simulink model "I_f_control_Rotor_pos_est"  (R2021b)
settings: Solver=FixedStepDiscrete  StartTime=0.0  StopTime=inf  RelTol=1e-3  EnableMultiTasking=on
model workspace (MAT data in the model file):
  samples = 1000
values from neighbouring files (symbols this model uses):
  alphac = 2*pi*300    (= 1884.95559215)    [init.m]
  Ls = 0.2e-3    (= 0.0002)    [init.m]
  max_rate = 100    [init.m]
  min_rate = -100    [init.m]
  p = 8    [Mtpa.m]    (also in init.m = 4)
  PositionOffset = 3.512    [init.m]
  psi_f = single((Ke)/(sqrt(3)*2*pi*1000*p/60))    [init.m]
  PWM_timer_period = (CPU_clock/Sys_clock_div/fsw/2)/4    (= 1250)    [init.m]
  Rs = 0.36    [init.m]
  Time_needed = Timeconstant*5    (= 0.00277777777778)    [init.m]
  Ts = 1/(4*fsw)    (= 2.5e-05)    [init.m]
undefined symbols (not defined in the file or in its folder): Down, GPTRIP1SEL, GPTRIP2SEL, TZ1, TZ2, Up
libraries: c2802xlib x7, c280xlib x3, c2837xDlib x3, mcbpositiondecoderlib x3, c2000lib x1, simulink x1
(part 2 of 2)

== matlab function I_f_control_Rotor_pos_est/Subsystem/Subsystem/MATLAB Function ==
  data: long_pulse input; wm input; estimator input; Rs input; Lq output; vd input; Ld output; vq input; id input; iq input; is_ref input; d_align input; start_pm_flux input; psi_d_old input; psi_d_new output; Ts parameter; Ld_old input; psi_q_old input; Lq_old input; vd_rs output; psi_q_new output; vq_rs output; vq_rs_old input; Time_needed parameter; Rs_delta_old input; Rs_delta output; vd_rs_old input; psi_PM output; stop output; Rs_new output
function [Lq,Ld,psi_d_new,vd_rs,psi_q_new,vq_rs,Rs_delta, psi_PM, stop, Rs_new] = fcn(long_pulse,wm,estimator,Rs,vd,vq,id,iq,is_ref,d_align, start_pm_flux,psi_d_old,Ts,Ld_old,psi_q_old,Lq_old,vq_rs_old,Time_needed,Rs_delta_old,vd_rs_old)

Lq = single(0);
Ld = single(0);
psi_d_new = psi_d_old;
psi_q_new = single(0);
persistent Rs_per
persistent pm_flux

if id>0.95*real(is_ref) && long_pulse==1
    stop=single(1);
elseif (d_align == 1 && real(is_ref) > 0)
    Rs=vd/id;%scetchy testing, star connection calc might be needed...
    Rs_per=Rs;
    stop=single(0);
else
    stop=single(0);
end
if isempty(Rs_per)
    Rs_new=single(0);
else
    Rs_new=single(Rs_per);
end

if isempty(Rs_per)
    psi_d = single(0);
    vd_rs = single(0); %Debug
    psi_q = single(0);
    vq_rs = single(0); %Debug
else
    psi_d = single((vd-Rs_per*id)*Ts);
    vd_rs = vd-Rs_per*id; %Debug
    psi_q = single((vq-Rs_per*iq)*Ts);
    vq_rs = vq-Rs_per*iq; %Debug
end

if imag(is_ref) > 0 
    vq_rs = vq-Rs*imag(is_ref); %Debug
    psi_q_new = single(psi_q+psi_q_old);
    Lq = psi_q_new/iq;
else
    vq_rs = vq_rs_old;
    psi_q_new = psi_q_old;
    Lq = Lq_old - vq_rs*(Time_needed);
    vq_rs =single(0);

end

% %For d-component
psi_d_new = single(0);
if  (real(is_ref) > 0 && estimator == 1 )
    %vd_rs = vd-Rs*id; %Debug
    Rs_delta = single(vd_rs/id);
    psi_d_new = single(psi_d+psi_d_old);
    Ld = psi_d_new/id;
else
    %vd_rs = vd_rs_old;
    Rs_delta = Rs_delta_old;
    psi_d_new = single(0);
    Ld = Ld_old; %- vd_rs*(Time_needed);
    %vd_rs = single(0);

end
if (start_pm_flux > 0)
    pm_flux = vq/wm;
end
if isempty(pm_flux)
    psi_PM=single(0);
else
    psi_PM=single(pm_flux *(1000*sqrt(2)));
end

== matlab function I_f_control_Rotor_pos_est/Subsystem/Subsystem5/MATLAB Function ==
  data: ThetaM input; ThetaM output; d_magnitize input; offset output; offset_old input
function [ThetaM, offset]  = fcn(ThetaM, d_magnitize, offset_old)


if d_magnitize == 1
    offset = ThetaM;
    ThetaM = single(0);
else
    offset = offset_old;
    ThetaM = ThetaM - offset;
end

== matlab function I_f_control_Rotor_pos_est/Subsystem/Subsystem2/MATLAB Function ==
  data: trigger output; pulseaxis output; sample_number output; long_pulse output; d_align output; start_pm_flux output; est input; stop input; c input; cnew output
function [trigger,pulseaxis,sample_number, long_pulse, d_align, start_pm_flux,cnew]= fcn(est,stop,c)

bool=single(0);
%Rs = single(0);
cnew=single(0);
long_pulse=single(0);
persistent sample
pulseaxis=single(1);
%sample_number=single(0);
if (est==1)
    cnew=c+1;
    if (cnew<45000) % d axis align
        bool=single(1);
        pulseaxis=single(1);
        sample_number=single(30000);
        d_align = single(1);
        start_pm_flux = single(0);
    
    elseif (cnew>45000 && cnew<65000) % check when reaching steady state
        bool=single(1);
        pulseaxis=single(1);
        sample_number=single(1000);
        long_pulse=single(1);
        d_align = single(0);
        start_pm_flux = single(0);
        if stop==1 && isempty(sample)
            sample=cnew-45000;
        end
    elseif (cnew>65000 && cnew<85000) % d pulse
        d_align = single(0);
        start_pm_flux = single(0);
        if isempty(sample)
            sample_number=single(0);
        else
            sample_number=single(sample);
            bool=single(1);
            pulseaxis=single(1);
        end
    elseif (cnew>85000 && cnew<100000) %q pulse
        d_align = single(0);
        start_pm_flux = single(0);
        if isempty(sample)
            sample_number=single(0);
        else
            sample_number=single(sample);
            bool=single(1);
            pulseaxis=single(0);
        end
    elseif (cnew>100000 && cnew<400000) %zeroing the counter if est kept on
        start_pm_flux = single(1000);
        sample_number=single(0);
        d_align = single(0);
    elseif (cnew>400000) %zeroing the counter if est kept on
        start_pm_flux = single(0);
        sample_number=single(0);
        d_align = single(0);
        cnew=cnew-1;
    else
        start_pm_flux = single(0);
        sample_number=single(0);
        d_align = single(0);
    end
    
else
    start_pm_flux = single(0);
    sample_number=single(0);
    d_align = single(0);
end

trigger=single(bool);

== matlab function I_f_control_Rotor_pos_est/Subsystem/Subsystem4/MATLAB Function2 ==
  data: is_ref output; axis input; trigger input; Sample_Number input; sample_time_new input; sample_time_old output
function [is_ref,sample_time_old] = fcn(axis,trigger,Sample_Number,sample_time_new)
id=0;
iq=0;
sample_number=single(0);
if (trigger == 1)
    if (sample_time_new < Sample_Number)
        sample_number=sample_time_new+1;
        if axis==0
            id=0;
            iq=1;
        elseif axis==1
            id=1;
            iq=0;
        else
            id=0;
            iq=0;
        end
    else 
        sample_number = sample_time_new;
    end
end
sample_time_old=sample_number;
is_ref=real(single(id))+imag(single(iq));

== matlab function I_f_control_Rotor_pos_est/Subsystem/If statement1/MATLAB Function ==
  data: is_ref_estimator input; is_ref_to_controller output; is_ref input; start input; d_magnatize input; d_mag input; start_pm_flux input; pm_flux_current input
function is_ref_to_controller = If_operation(is_ref_estimator,is_ref, start, d_magnatize, d_mag, start_pm_flux, pm_flux_current)

if start > 0
    is_ref_to_controller = is_ref;
elseif d_magnatize > 0
    is_ref_to_controller = d_mag;
elseif start_pm_flux > 0
    is_ref_to_controller =  pm_flux_current;
else
    is_ref_to_controller = is_ref_estimator;

end

== matlab function I_f_control_Rotor_pos_est/Subsystem/Current Controller and PWM/MATLAB Function1 ==
  data: is_ref input size=1; is input size=1; ws input; thetas input size=1; Udc input size=1; I input size=1; Rs parameter; Ls parameter size=1; alphac parameter size=1; Ts parameter size=1; d_abc output size=3; us_ref output; Inew output; psi_f parameter; enable input
function [d_abc,us_ref, Inew] = cc(is_ref, is, ws, thetas, Udc, I, Rs, Ls, alphac, Ts, psi_f, enable)
%#codegen


%% Current controller 
% Gains
kp = alphac*Ls;
ki = alphac^2*Ls;
Ra = alphac*Ls - Rs;

% Voltage reference in synchronous coordinates
e = is_ref - is;
us_ref = kp*e + ki*I - Ra*is + 1j*ws*(Ls*is + psi_f);

    
% Reference in stator coordinates
thetasc = thetas + 1.5*Ts*ws;   % Compensation for discrete-time delays
if (enable == 1) 
uss_ref = us_ref*exp(1j*thetasc);
else 
    uss_ref = single(0 + 0*1j);
end

%% Symmetrical suboscillation PWM
% Components of the voltage space vector
ualpha_ref = real(uss_ref);
ubeta_ref  = imag(uss_ref);

% Phase-voltage references
ua_ref = ualpha_ref;
ub_ref = .5*(-ualpha_ref + sqrt(3)*ubeta_ref);
uc_ref = .5*(-ualpha_ref - sqrt(3)*ubeta_ref);

% Vector of phase-voltage references
u_abc_ref = [ua_ref; ub_ref; uc_ref];

% Symmetrization of the references by adding the zero-sequence voltage
u0 = .5*(max(u_abc_ref) + min(u_abc_ref));
u_abc_ref = u_abc_ref - u0;

% Clamping of the reference voltages such that no phase error is caused. 
% If all phase voltage reference are realizable (below Udc/2), m = 1 holds.
m = max([2*u_abc_ref/Udc; 1]);
u_abc_ref = u_abc_ref/m;

% Duty cycles, which can be directly used for triangle comparison, 
% if the triangle wave varies between 0...1
d_abc = single(.5 + u_abc_ref/Udc);
% end
% Realized voltage vector is calculated from the clamped duty ratios.
% If the PWM does not saturate, us_ref_lim = us_ref holds. The realized
% voltage vector is needed, e.g., for the current-controller antiwindup.
uss_ref_lim = single(2/3*(d_abc(1) + d_abc(2)*exp(1j*2*pi/3) + d_abc(3)*exp(1j*4*pi/3))*Udc);
% In estimated rotor flux coordinates
us_ref_lim = single(exp(-1j*thetasc)*uss_ref_lim);  

%% Update the integral state of the current controller 
if (enable == 1) 
Inew = single(I + Ts*(e + (us_ref_lim - us_ref)/kp));
else 
    Inew = single(0+0*1j);
end

== matlab function I_f_control_Rotor_pos_est/Subsystem/Integrator ==
  data: Ts parameter; w_ref input; theta_new output single; theta input
function theta_new  = fcn(Ts, w_ref,theta)

theta_new = theta + Ts*w_ref;

% Limit the angle between [-pi,pi]
while(theta_new > pi)
    theta_new = theta_new - 2*pi;
end
while(theta_new < -pi) 
    theta_new = theta_new + 2*pi;
end

== matlab function I_f_control_Rotor_pos_est/Subsystem/Protection /Protection ==
  data: Udc input; fault output; Idc input; Umin input; Umax input; Imax input; reset input; start input; run_enable input; prev_fault_state input
function fault = protection(Udc, Idc, Umin, Umax, Imax, reset, start, run_enable, prev_fault_state)
if (Udc < Umin || Udc > Umax || Idc > Imax)   
    fault = single(1);
else
    fault = prev_fault_state;
end

if (reset == 1 && fault == 1 && start == 0 && run_enable == 0)
   fault = single(0);
end

== matlab function I_f_control_Rotor_pos_est/Subsystem/Rate limiter ==
  data: estimate input; in input single; run_enable input; out input; out output; max_rate parameter; min_rate parameter; Ts parameter
function out  = fcn(estimate, in, run_enable, out, max_rate, min_rate, Ts)
if run_enable == 0
    out = single(0);
elseif(estimate > 0)
    in = estimate * (2*pi/60);
end

persistent rate
        
    if isempty(rate)
        rate = (in-out)/Ts;
    else
    rate = (in-out)/Ts;
    end
    if (rate > max_rate)
        out = Ts*max_rate + out;
    elseif (rate < min_rate)
        out = Ts*min_rate + out;
    elseif (rate > min_rate || rate < max_rate)
        out = in;
    end

== matlab function I_f_control_Rotor_pos_est/Subsystem/Subsystem1/1st order filter ==
  data: in input; y output; y_prev input; a parameter
function y = filter(in, y_prev, a)

y = (1-a)*y_prev + in*a;
